simulink model "variantAndSubsystemRefTest"  (R2023b)
settings: Solver=VariableStepAuto  StartTime=0.0  StopTime=10.0  RelTol=1e-3
settings Model: Creator=pkesarwa  LastModifiedBy=pkesarwa

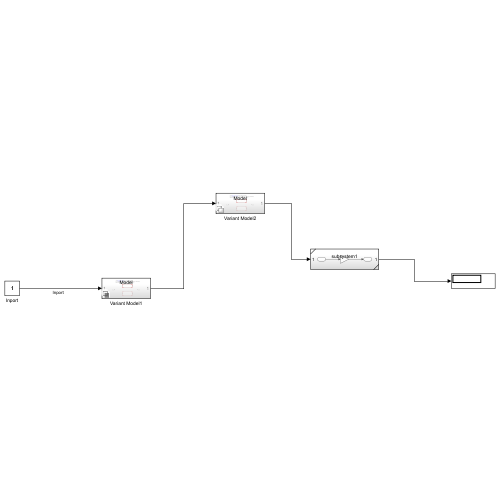
[thumbnail: Simulink's stored preview of the top-level diagram]
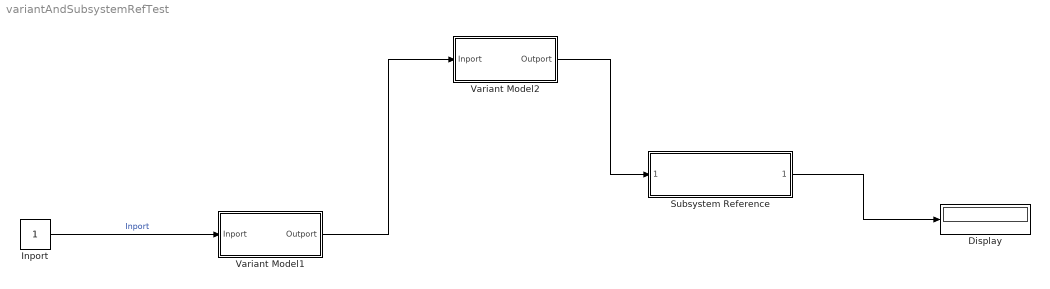
== system variantAndSubsystemRefTest ==
  Display : Display
  Inport : Constant
  Subsystem Reference : Subsystem  ReferencedSubsystem=subsystem1
  Variant Model1 : Subsystem  Variant=on  VariantControlMode=label  LabelModeActiveChoice=one
  Variant Model2 : Subsystem  Variant=on
  wires:
  Inport/1 -> Variant Model1/1(Inport)  "Inport"
  Variant Model1/1(Outport) -> Variant Model2/1(Inport)
  Variant Model2/1(Outport) -> Subsystem Reference/1
  Subsystem Reference/1 -> Display/1

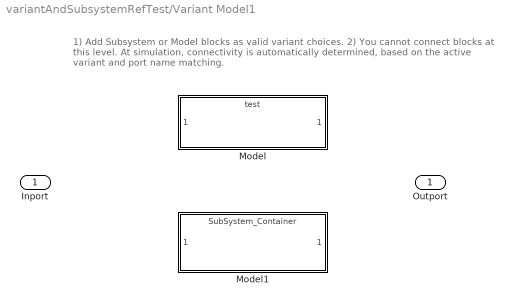
== system variantAndSubsystemRefTest/Variant Model1 ==
  note: 1) Add Subsystem or Model blocks as valid variant choices.
      | 2) You cannot connect blocks at this level. At simulation, connectivity is automatically
      | determined, based on the active variant and port name matching.
  Inport : Inport
  Model : ModelReference  DisableCoverage=on  ModelNameDialog=test.slx  VariantControl=one  ModelReferenceVersion=3.1
  Model1 : ModelReference  ModelNameDialog=SubSystem_Container.slx  VariantControl=two  ModelReferenceVersion=1.3
  Outport : Outport

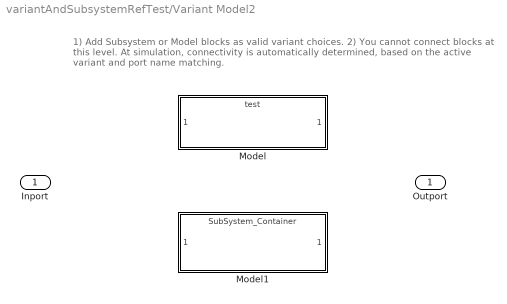
== system variantAndSubsystemRefTest/Variant Model2 ==
  note: 1) Add Subsystem or Model blocks as valid variant choices.
      | 2) You cannot connect blocks at this level. At simulation, connectivity is automatically
      | determined, based on the active variant and port name matching.
  Inport : Inport
  Model : ModelReference  DisableCoverage=on  ModelNameDialog=test.slx  VariantControl=true  ModelReferenceVersion=3.1
  Model1 : ModelReference  ModelNameDialog=SubSystem_Container.slx  VariantControl=false  ModelReferenceVersion=1.3
  Outport : Outport
